simulink model "ant_spring_ctrl"  (R2023a)
settings: Solver=ode4  StartTime=0.0  StopTime=60  FixedStep=0.001  RelTol=1e-3
model workspace (MAT data in the model file):
  a_mdh = [0.5; 0.5]
  alpha_mdh = [0; 0]
  d_mdh = [0; 0]
  l0 = [0.189353021319; 0.189353021319; 0.583222456778; 0.583222456778; 0.682071526229; 0.682071526229]
  p1_sol = [-196.46190846; -196.46190846; -196.46190846; -196.46190846; -196.46190846; 244.7265907; 244.7265907; 244.7265907; 244.7265907; 244.7265907; 0.108119886166; 0.108119886166; 0.108119886166; 0.108119886166; 0.108119886166]
  p2_sol = [-39.726939819; -163.425908656; -189.145615997; -193.604265592; -219.559697571; 44.5746374772; 153.533472233; 68.0096135047; 63.0706600389; 365.58131095; 0.927523422495; 0.37135489076; 0.295363504694; 0.295780130224; 0.415380975864]
  p3_sol = [-152.907364382; -153.38439627; -153.384182952; -153.387392656; -153.387514498; 82.883192474; 156.637043328; 156.637072219; 156.662654025; 156.665094103; 0.0711552458823; 0.16264087768; 0.162640870132; 0.162634189747; 0.16263355254]
values from neighbouring files (symbols this model uses):
  period = 5    [dynamics_n_dof_c.m]
  RR = randrot(3,2)    [dynamics_n_dof_c.m]
libraries: commrandsrc3 x2, simulink x1
settings Model: Creator=dennis  LastModifiedBy=diaz
settings SolverCC: AlgebraicLoopSolver=TrustRegion
settings DebuggingCC: UnconnectedInputMsg=warning  UnconnectedOutputMsg=warning  UnconnectedLineMsg=warning
settings ModelReferenceCC: EnableRefExpFcnMdlSchedulingChecks=on
settings RTWCC: DLArmComputeVersion=19.05

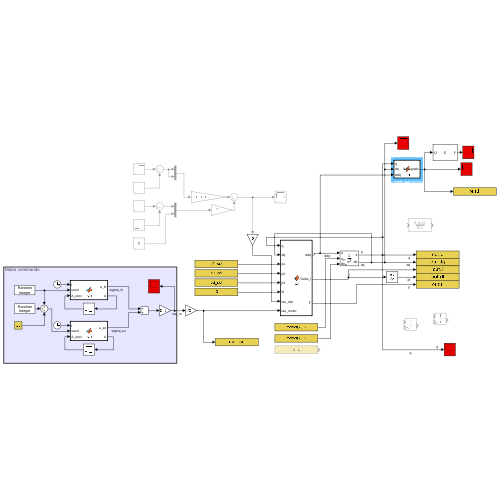
[thumbnail: Simulink's stored preview of the top-level diagram]
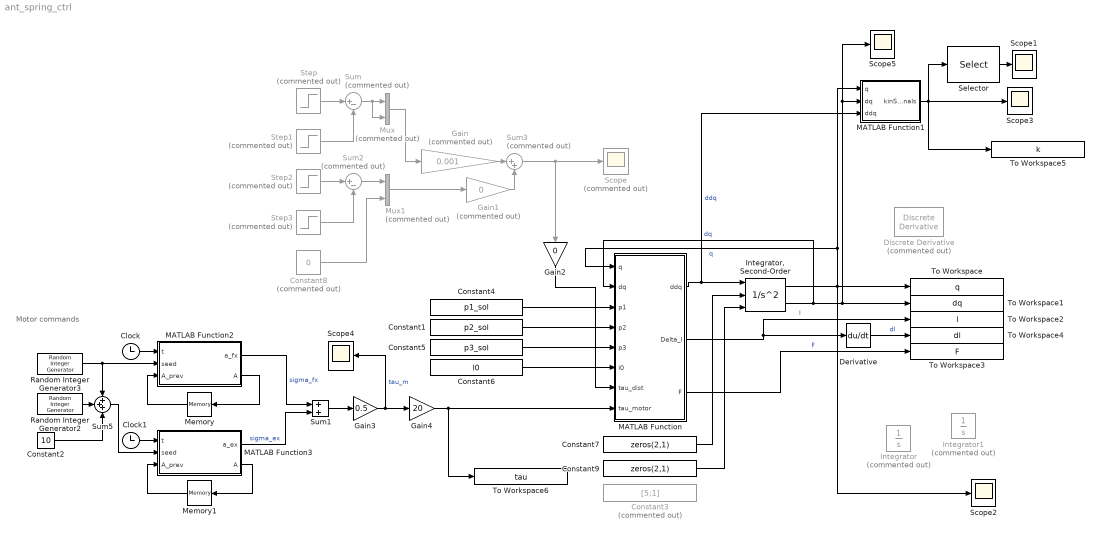
== system ant_spring_ctrl ==
  note: Motor commands
  Clock : Clock
  Clock1 : Clock
  Constant1 : Constant  Value=p2_sol
  Constant2 : Constant  Value=10
  Constant3 : Constant  Commented=on  Value=[5;1]
  Constant4 : Constant  Value=p1_sol
  Constant5 : Constant  Value=p3_sol
  Constant6 : Constant  Value=l0
  Constant7 : Constant  Value=zeros(2,1)
  Constant8 : Constant  Commented=on  Value=0
  Constant9 : Constant  Value=zeros(2,1)
  Derivative : Derivative
  Discrete Derivative : simulink/Discrete/Discrete Derivative  Commented=on  gainval=1.0  ICPrevScaledInput=0.0  OutMin=[]  OutMax=[]  OutDataType=fixdt(1, 16)  OutScaling=2^-10  DoSatur=off
  Gain : Gain  Commented=on  Gain=0.001
  Gain1 : Gain  Commented=on  Gain=0
  Gain2 : Gain  Gain=0
  Gain3 : Gain  Gain=0.5
  Gain4 : Gain  Gain=20
  Integrator : Integrator  Commented=on  InitialConditionSource=external
  "Integrator, Second-Order" : SecondOrderIntegrator  ICSourceX=external  ICSourceDXDT=external
  Integrator1 : Integrator  Commented=on  InitialConditionSource=external
  MATLAB Function : MATLAB Function  TreatAsAtomicUnit=on
  MATLAB Function1 : MATLAB Function  TreatAsAtomicUnit=on
  MATLAB Function2 : MATLAB Function  TreatAsAtomicUnit=on
  MATLAB Function3 : MATLAB Function  TreatAsAtomicUnit=on
  Memory : Memory  InitialCondition=zeros(2,3)
  Memory1 : Memory  InitialCondition=zeros(2,3)
  Mux : Mux  Commented=on  Inputs=2
  Mux1 : Mux  Commented=on  Inputs=2
  Random Integer Generator2 : commrandsrc3/Random Integer Generator  SetSize=period  SeedSource=Auto  Seed=0  SampleTime=1  SamplesPerFrame=1  OutputDataType=double  SimulateUsing=Interpreted execution
  Random Integer Generator3 : commrandsrc3/Random Integer Generator  SetSize=10  SeedSource=Auto  Seed=0  SampleTime=period  SamplesPerFrame=1  OutputDataType=double  SimulateUsing=Interpreted execution
  Scope : Scope  Commented=on
  Scope{1..5} (5 alike) : Scope
  Selector : Selector  InputPortWidth=27  IndexOptions=Index vector (dialog)  Indices=[19:27]  OutputSizes=1
  Step : Step  Commented=on  SampleTime=0
  Step1 : Step  Commented=on  Time=1.1  SampleTime=0
  Step2 : Step  Commented=on  Time=10  SampleTime=0
  Step3 : Step  Commented=on  Time=10.1  SampleTime=0
  Sum : Sum  Commented=on  Inputs=|+-
  Sum1 : Sum
  Sum2 : Sum  Commented=on  Inputs=|+-
  Sum3 : Sum  Commented=on  Inputs=|++
  Sum5 : Sum  Inputs=+++
  To Workspace : ToWorkspace  VariableName=q  SaveFormat=Timeseries  SampleTime=-1
  To Workspace1 : ToWorkspace  VariableName=dq  SaveFormat=Timeseries  SampleTime=-1
  To Workspace2 : ToWorkspace  VariableName=l  SaveFormat=Timeseries  SampleTime=-1
  To Workspace3 : ToWorkspace  VariableName=F  SaveFormat=Timeseries  SampleTime=-1
  To Workspace4 : ToWorkspace  VariableName=dl  SaveFormat=Timeseries  SampleTime=-1
  To Workspace5 : ToWorkspace  VariableName=k  SaveFormat=Timeseries  SampleTime=-1
  To Workspace6 : ToWorkspace  VariableName=tau  SaveFormat=Timeseries  SampleTime=-1
  wires:
  MATLAB Function/1(ddq) -> MATLAB Function1/3(ddq), "Integrator, Second-Order"/1  "ddq"
  "Integrator, Second-Order"/1 -> MATLAB Function1/1(q), MATLAB Function/1(q), To Workspace/1, Scope2/1  "q"
  Constant1/1 -> MATLAB Function/4(p2)
  Constant7/1 -> "Integrator, Second-Order"/2
  "Integrator, Second-Order"/2 -> MATLAB Function/2(dq), Scope5/1, MATLAB Function1/2(dq), To Workspace1/1  "dq"
  Constant9/1 -> "Integrator, Second-Order"/3
  Mux/1 -> Gain/1
  Sum/1 -> Mux/2, Mux/1
  Step/1 -> Sum/1
  Step1/1 -> Sum/2
  Sum2/1 -> Mux1/1
  Step3/1 -> Sum2/2
  Step2/1 -> Sum2/1
  Gain/1 -> Sum3/1
  Sum3/1 -> Gain2/1, Scope/1
  Mux1/1 -> Gain1/1
  Gain1/1 -> Sum3/2
  Constant8/1 -> Mux1/2
  Constant4/1 -> MATLAB Function/3(p1)
  Constant5/1 -> MATLAB Function/5(p3)
  Constant6/1 -> MATLAB Function/6(l0)
  Gain2/1 -> MATLAB Function/7(tau_dist)
  MATLAB Function/2(Delta_l) -> Derivative/1, To Workspace2/1  "l"
  MATLAB Function/3(F) -> To Workspace3/1  "F"
  Derivative/1 -> To Workspace4/1  "dl"
  MATLAB Function1/1(kinSignals) -> Selector/1, To Workspace5/1, Scope3/1
  Memory/1 -> MATLAB Function2/3(A_prev)
  Clock/1 -> MATLAB Function2/1(t)
  MATLAB Function3/1(a_ex) -> Sum1/2  "sigma_ex"
  Constant2/1 -> Sum5/3
  MATLAB Function3/2(A) -> Memory1/1
  MATLAB Function2/2(A) -> Memory/1
  Random Integer Generator2/1 -> Sum5/2
  Sum5/1 -> MATLAB Function3/2(seed)
  Memory1/1 -> MATLAB Function3/3(A_prev)
  Clock1/1 -> MATLAB Function3/1(t)
  Random Integer Generator3/1 -> Sum5/1, MATLAB Function2/2(seed)
  MATLAB Function2/1(a_fx) -> Sum1/1  "sigma_fx"
  Gain3/1 -> Gain4/1, Scope4/1  "tau_m"
  Sum1/1 -> Gain3/1
  Gain4/1 -> To Workspace6/1, MATLAB Function/8(tau_motor)
  Selector/1 -> Scope1/1

== matlab function ant_spring_ctrl/MATLAB Function1 ==
  data: q input; kinSignals output; dq input; ddq input; a_mdh parameter; RR parameter
function kinSignals   = fcn(q, dq, ddq, a_mdh, RR)

z_vec = [0;0;1];

% angVel_0_in_0 = zeros(3,1);
% lin_vel_0_in_0 = zeros(3,1);
% 
% ang_Acc_0_in_0 = zeros(3,1);
% lin_Acc_0_in_0 = zeros(3,1);
% 
% p_0_to_1  = [0;0;0];
% p_1_to_2  = [a_mdh(1);0;0];
% p_1_to_s1 = [0.2;0;0];



i_p_j  = [0,0,0;
          a_mdh(1),0,0]';

j_p_sj  = [0.2,0,0;
           0.35,0,0]';

angVel = zeros(3,3);
% LinVel = zeros(3,3);
angAcc = zeros(3,3);
linAcc = zeros(3,3);

sensorAngVel = zeros(3,3);
% sensorLinVel = zeros(3,3);
sensorAngAcc = zeros(3,3);
sensorLinAcc = zeros(3,3);

for j = (1:2)+1
    j_R_i                 = transpose(rotz(q(j-1)));
    s_R_j                 = RR(:,:,j-1);
    i_Omg_i               = angVel(:,j-1);
    i_dOmg_i              = angAcc(:,j-1);
    i_dVel_i              = linAcc(:,j-1);

    angVel(:,j)       = j_R_i*i_Omg_i + dq(j-1)*z_vec;
    sensorAngVel(:,j) = s_R_j*angVel(:,j);
    
    angAcc(:,j)       = j_R_i*i_dOmg_i + skew(j_R_i*i_Omg_i)*dq(j-1)*z_vec + ddq(j-1)*z_vec;
    sensorAngAcc(:,j) = s_R_j*angAcc(:,j);
    
    linAcc(:,j)       = j_R_i*(i_dVel_i + skew(i_dOmg_i)*i_p_j(:,j-1) + skew(i_Omg_i)*skew(i_Omg_i)*i_p_j(:,j-1));
                             % j_dVel_j + skew(j_dOmg_j)*j_p_s(:,j-1) + skew(j_Omg_j)*skew(j_Omg_j)*j_p_s(:,j-1); 
    sensorLinAcc(:,j) = s_R_j*(linAcc(:,j) + skew(angAcc(:,j))*j_p_sj(:,j-1) + skew(angVel(:,j))*skew(angVel(:,j))*j_p_sj(:,j-1)); 
end

kinSignals = [sensorAngVel(:);
              sensorAngAcc(:);
              sensorLinAcc(:)];


% R_0_to_1     = transpose(rotz(q(1)));
% Omg_1_in_1   = R_0_to_1*angVel_0_in_0 + dq(1)*z_vec;
% Omg_s1_in_s1 = RR(:,:,1)*Omg_1_in_1;
% Vel_1_in_1   = R_0_to_1*(lin_vel_0_in_0 + skew(angVel_0_in_0)*p_0_to_1);
% %Vel_1_s1  = Vel_1_1 + skew(Omg_1_1)*[0.2;0;0];
% %Vel_s1_s1 = RR(:,:,1)*Vel_1_s1;
% 
% dOmg_1_in_1   = R_0_to_1*ang_Acc_0_in_0 + skew(R_0_to_1*angVel_0_in_0)*dq(1)*z_vec + ddq(1)*z_vec;
% dOmg_s1_in_s1 = RR(:,:,1)*dOmg_1_in_1;
% dVel_1_in_1   = R_0_to_1*(skew(ang_Acc_0_in_0)*p_0_to_1 + skew(angVel_0_in_0)*skew(angVel_0_in_0)*p_0_to_1 + lin_Acc_0_in_0);
% dVel_1_in_s1  = dVel_1_in_1 + skew(dOmg_1_in_1)*p_1_to_s1 + skew(Omg_1_in_1)*skew(Omg_1_in_1)*p_1_to_s1; 
% dVel_s1_in_s1 = RR(:,:,1)*dVel_1_in_s1;
% 
% R_1_to_2  = transpose(rotz(q(2)));
% Omg_2_2   = R_1_to_2*Omg_1_in_1 + dq(2)*[0;0;1];
% Omg_s2_s2 = RR(:,:,2)*Omg_2_2;
% Vel_2_2   = R_1_to_2*(Vel_1_in_1 + skew(Omg_1_in_1)*[a_mdh(1);0;0]);
% %Vel_2_s2  = Vel_2_2 + skew(Omg_2_2)*[0.35;0;0];
% %Vel_s2_s2 = RR(:,:,2)*Vel_2_s2;
% 
% dOmg_2_2   = R_1_to_2*dOmg_1_in_1 + skew(R_1_to_2*angVel_0_in_0)*dq(2)*z_vec + ddq(2)*z_vec;
% dOmg_s2_s2 = RR(:,:,2)*dOmg_2_2;
% dVel_2_2   = R_1_to_2*(skew(dOmg_1_in_1)*[a_mdh(1);0;0] + skew(Omg_1_in_1)*skew(Omg_1_in_1)*[a_mdh(1);0;0] + dVel_1_in_1);
% dVel_2_s2  = dVel_2_2 + skew(dOmg_2_2)*[0.35;0;0] + skew(Omg_2_2)*skew(Omg_2_2)*[0.35;0;0]; 
% dVel_s2_s2 = RR(:,:,2)*dVel_2_s2;
% 
% nu = [Omg_1_in_1, Omg_2_2;
%       Vel_1_in_1, Vel_2_2];
% 
% dnu = [dOmg_1_in_1, dOmg_2_2;
%        dVel_1_in_1, dVel_2_2];
% 
% kinSignals = [Omg_s1_in_s1;dOmg_s1_in_s1;dVel_s1_in_s1;...
%               Omg_s2_s2;dOmg_s2_s2;dVel_s2_s2];



end

== matlab function ant_spring_ctrl/MATLAB Function ==
  data: q input; dq input; p1 input; ddq output; p2 input; p3 input; l0 input; tau_dist input; Delta_l output; F output; tau_motor input
function [ddq, Delta_l, F] = fcn(q, dq, p1, p2, p3, l0, tau_dist, tau_motor)


C       = get_C(q,dq);
%G = get_G(q);
M       = get_M(q);
%l0 = get_l(zeros(2,1));
n_w     = 5;
l       = get_l(q);
Delta_l = l0 - l;

% Spring forces
F= [...
    rbf_sym(Delta_l(1), p1(1:n_w),p1(n_w+1:2*n_w),p1(2*n_w+1:3*n_w));
    rbf_sym(Delta_l(2), p1(1:n_w),p1(n_w+1:2*n_w),p1(2*n_w+1:3*n_w));
    rbf_sym(Delta_l(3), p2(1:n_w),p2(n_w+1:2*n_w),p2(2*n_w+1:3*n_w));
    rbf_sym(Delta_l(4), p2(1:n_w),p2(n_w+1:2*n_w),p2(2*n_w+1:3*n_w));
    rbf_sym(Delta_l(5), p3(1:n_w),p3(n_w+1:2*n_w),p3(2*n_w+1:3*n_w));
    rbf_sym(Delta_l(6), p3(1:n_w),p3(n_w+1:2*n_w),p3(2*n_w+1:3*n_w))...
    ];
%%
q1 = q(1);
q2 = q(2);
l = 0.5;

Jy = [- l*sin(q1 + q2) - l*sin(q1), -l*sin(q1 + q2)];
Jx = [  l*cos(q1 + q2) + l*cos(q1),  l*cos(q1 + q2)];

%%
K      = 75* get_M(q);
disp   = (deg2rad([40; -80]) - q);
tau_cc = K * disp;


U  = 0.5 * disp' * K * disp;
T  = 0.5 * dq'*M*dq;
H  = U + T;
Hd = 10;

q1 = q(1); q2 = q(2);
l = 0.5;
Jx = [- l*sin(q1 + q2) - l*sin(q1), -l*sin(q1 + q2)];
Jy = [  l*cos(q1 + q2) + l*cos(q1),  l*cos(q1 + q2)];

tau_in =  -50 * Jy' * (Jy* dq) ;
%tau_in = tau_in + 10*x_gain * Jx' * (Jx* dq);


tau_in = tau_in + 1*(Hd-H) * Jx' * (Jx* dq);
%%

tau_springs = get_tau_F(q,F) ;

ddq = M\(tau_springs + tau_dist - C*dq + tau_motor);

end

== matlab function ant_spring_ctrl/MATLAB Function2 ==
  settings: updateMethod=DISCRETE  sampleTime=1E-3
  data: t input; seed input; a_fx output; A_prev input; period parameter; A output
function [a_fx, A]  = fcn(t, seed, A_prev, period)
    a =-1;
    b = 1;
    rng(1)
    
    if mod(t, period ) == 0
        rng(seed)
        A_base = rand(2,3);
        A      = (b-a).*A_base + a; 
    else
        A = A_prev;
    end
    
    for j=1:2        
        A(j,:) = A(j,:);%./sum(abs(A(j,:))); 
    end
        
    sinusoids = [sin(2*pi/period*t);
                 sin(2*pi/(0.5*period)*t);
                 sin(2*pi/(0.25*period)*t)];
    
    a_fx = tanh(A*sinusoids); 

end

== matlab function ant_spring_ctrl/MATLAB Function3 ==
  settings: updateMethod=DISCRETE  sampleTime=1E-3
  data: t input; seed input; a_ex output; A_prev input; A output; period parameter
function [a_ex,A] = fcn(t, seed, A_prev, period)
a =-1;
b = 1;
rng(1)
% sigmoid = @(x,a) 1./(1 + exp(-a*(x)));
% period           = 5;

if mod(t, period ) == 0
    rng(seed)
    A_base = rand(2,3);
    A      = (b-a).*A_base + a; 
else
    A = A_prev;
end

for j=1:2
    A(j,:) = A(j,:);%./sum(abs(A(j,:))); 
end
    
sinusoids = [sin(2*pi/period*t);
             sin(2*pi/(0.5*period)*t);
             sin(2*pi/(0.25*period)*t)];


a_ex  = tanh(A*sinusoids);
